simulink model "guidance"  (R2021a)
settings: Solver=VariableStepAuto  StartTime=0.0  StopTime=inf  RelTol=1e-3
values from neighbouring files (symbols this model uses):
  A_mpc = blkdiag([1 dt 0;0 1 dt;0 0 1],[1 dt 0;0 1 dt;0 0 1],[1 dt 0;0 1 dt;0 0 1])    [init.m]
  B_mpc = zeros(9,3)    [init.m]
  C_mpc = [1 zeros(1,8);0 0 0 1 zeros(1,5); zeros(1,6) 1 0 0 ... (first row only)    [init.m]
  D_mpc = zeros(9,3)    [init.m]
  M = 1.5    [InitMain.m]    (also in init.m)
  wait = 5    [init.m]
libraries: mpclib x1, drivingscenarioandsensors x1
settings Model: Creator=Adam  LastModifiedBy=Adam

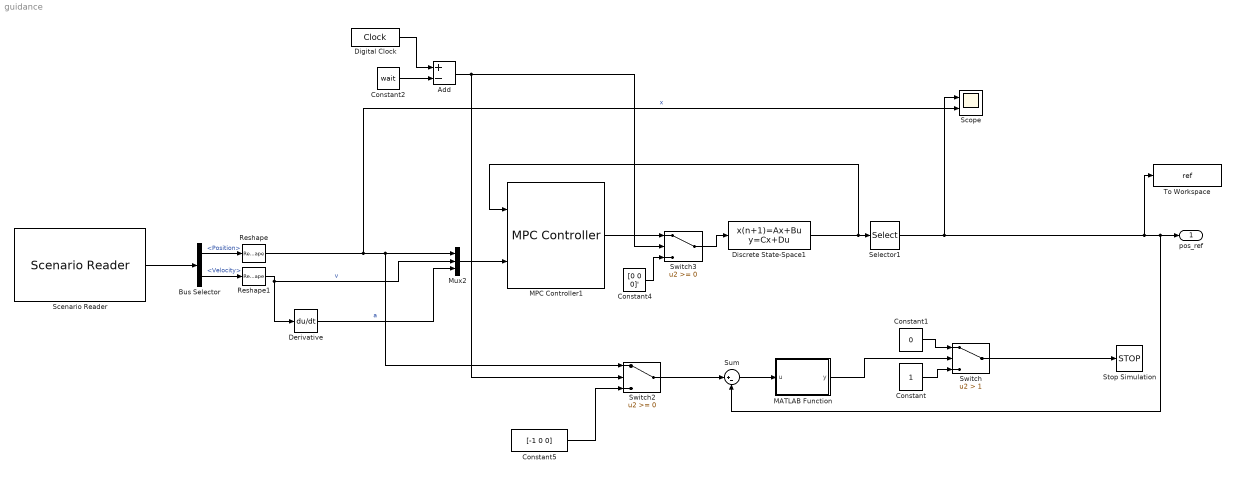
== system guidance ==
  Add : Sum  Inputs=+-
  Bus Selector : BusSelector  OutputSignals=Actors.Position,Actors.Velocity
  Constant : Constant
  Constant1 : Constant  Value=0
  Constant2 : Constant  Value=wait
  Constant4 : Constant  Value=[0 0 0]'
  Constant5 : Constant  Value=[-1 0 0]
  Derivative : Derivative
  Digital Clock : DigitalClock  SampleTime=0.01
  Discrete State-Space1 : DiscreteStateSpace  A=A_mpc  B=B_mpc  C=C_mpc  D=D_mpc  InitialCondition="[0;0;0; 0;0;0  ; 5 ;0;0]"  SampleTime=0.01
  MATLAB Function : MATLAB Function  TreatAsAtomicUnit=on
  MPC Controller1 : mpclib/MPC Controller  SCDEnableBlockLinearizationSpecification=on  is_multiple=0  enable_value=0  return_u0=off  updateMPCinCallerWorkspace=on  md_inport=off  mv_inport=off  uref_inport=off  return_cost=off  return_mvseq=off  return_qpstatus=off  return_xseq=off  return_state=off  return_ovseq=off  state_inport=off  umin_inport=off  umax_inport=off  ymin_inport=off  ymax_inport=off  cc_inport=off  ywt_inport=off  uwt_inport=off  duwt_inport=off  rhoeps_inport=off  pm_inport=off  MaximumP=10  HorizonChoice=FixedHorizon  n_ts=0.01  n_p=10  n_mv=3  n_md=0  n_ud=0  n_mo=9  n_uo=0  BlockDataType=double  SampleTimeInherited=off  switch_inport=off
  Mux2 : Mux  Inputs=3
  Reshape : Reshape
  Reshape1 : Reshape
  Scenario Reader : drivingscenarioandsensors/Scenario Reader  ScenarioSource=From file  ScenarioFileName=C:\Users\Adam\OneDrive\Desktop\M.Sc_LRT\4.sem\session2\Stage\sim\sc10m.mat  ScenarioVariableName=scenario  OutputCoordinateSystem=World coordinates  EgoVehicleSource=Scenario  EgoVehicleActorID=1  OrientVehiclesOnRoad=off  OutputEgoVehiclePose=off  SampleTime=0.01  LaneBoundaryOutput=None  LaneBoundaryDistance=0:0.5:9.5  LaneBoundaryLocation=Center of lane markings  BusNameSource=Auto  BusName=BusActors  BusNumActorsSource=Scenario  BusNumActors=100  BusName2Source=Auto  BusName2=BusLaneBoundaries  BusNumLaneBoundariesSource=Scenario  BusNumLaneBoundaries=10  BusName3Source=Auto  BusName3=BusEgoActor  ShowCoordinateLabels=on  SimulateUsing=Interpreted execution
  Scope : Scope  NumInputPorts=2
  Selector1 : Selector  InputPortWidth=9  IndexOptions=Index vector (dialog)  Indices=[1 2 3]  OutputSizes=1
  Stop Simulation : Stop
  Sum : Sum  Inputs=|+-
  Switch : Switch  Criteria=u2 > Threshold  Threshold=1
  Switch2 : Switch
  Switch3 : Switch
  To Workspace : ToWorkspace  VariableName=ref  SampleTime=-1
  pos_ref : Outport
  wires:
  Selector1/1 -> Scope/1, To Workspace/1, Sum/2, pos_ref/1
  Switch/1 -> Stop Simulation/1
  Sum/1 -> MATLAB Function/1(u)
  Constant1/1 -> Switch/1
  MATLAB Function/1(y) -> Switch/2
  Constant/1 -> Switch/3
  Discrete State-Space1/1 -> MPC Controller1/1, Selector1/1
  Mux2/1 -> MPC Controller1/2
  Scenario Reader/1 -> Bus Selector/1
  Bus Selector/1 -> Reshape/1  "<Position>"
  Derivative/1 -> Mux2/3  "a"
  Bus Selector/2 -> Reshape1/1  "<Velocity>"
  Reshape1/1 -> Mux2/2, Derivative/1  "v"
  Digital Clock/1 -> Add/1
  Constant2/1 -> Add/2
  Add/1 -> Switch2/2, Switch3/2
  Constant4/1 -> Switch3/3
  MPC Controller1/1 -> Switch3/1
  Switch3/1 -> Discrete State-Space1/1
  Switch2/1 -> Sum/1
  Reshape/1 -> Scope/2, Switch2/1, Mux2/1  "x"
  Constant5/1 -> Switch2/3

== matlab function guidance/MATLAB Function ==
  data: u input; y output
function y = fcn(u)

y = norm(u);
